simulink model "ForceBasedRollCenterVehicleModel"  (R2021b)
settings: Solver=VariableStepAuto  StartTime=0.0  StopTime=10.0  RelTol=1e-3
values from neighbouring files (symbols this model uses):
  AirDensity = 1.225    [PlanarModelWrapperScriptAttempt2.m]
  CoG = [(0.47-0.5)*Wheelbase, 0, 0.25]    [ForceBasedRollCenterModelWrapperScript.m]    (also in PlanarModelWrapperScriptAttempt2.m)
  CoP = [(0.4-0.5)*Wheelbase, 0, 0]    [PlanarModelWrapperScriptAttempt2.m]
  DragCoeff = 0.6    [PlanarModelWrapperScriptAttempt2.m]
  Front_Roll_Stiffness = 0    [ForceBasedRollCenterModelWrapperScript.m]
  Idx = 1    [3DOF Launch ControlHoosier_R25B_clean.mat]    (also in PlanarModelWrapperScriptAttempt2.m)
  Inclination = 1    [3DOF Launch ControlHoosier_R25B_clean.mat]    (also in PlanarModelWrapperScriptAttempt2.m)
  LiftCoeff = -1.9    [PlanarModelWrapperScriptAttempt2.m]
  Mass = 275    [ForceBasedRollCenterModelWrapperScript.m]    (also in PlanarModelWrapperScriptAttempt2.m)
  Model =     [3DOF Launch ControlHoosier_R25B_clean.mat]    (also in PlanarModelWrapperScriptAttempt2.m = struct( 'Pure', 'Pacejka', 'Combined', 'MNC' ))
  PercentFront = 0.5    [ForceBasedRollCenterModelWrapperScript.m]    (also in PlanarModelWrapperScriptAttempt2.m)
  PerLLT = 0.6    [PlanarModelWrapperScriptAttempt2.m]
  Pressure = 70    [3DOF Launch ControlHoosier_R25B_clean.mat]    (also in PlanarModelWrapperScriptAttempt2.m = 80)
  Rear_Roll_Stiffness = 0    [ForceBasedRollCenterModelWrapperScript.m]
  RefArea = 1.1    [PlanarModelWrapperScriptAttempt2.m]
  Roll_Dampening_Coeff_Front = 0    [ForceBasedRollCenterModelWrapperScript.m]
  Roll_Dampening_Coeff_Rear = 0    [ForceBasedRollCenterModelWrapperScript.m]
  Sprung_COG_Height = 0    [ForceBasedRollCenterModelWrapperScript.m]
  Tire =     [3DOF Launch ControlHoosier_R25B_clean.mat]
  TrackWidth = 1.22    [ForceBasedRollCenterModelWrapperScript.m]    (also in PlanarModelWrapperScriptAttempt2.m = 1.22*ones(1,2))
  TrackWidthTest = 1.22*ones(1,2)    [ForceBasedRollCenterModelWrapperScript.m]
  Wheelbase = 1.575    [ForceBasedRollCenterModelWrapperScript.m]    (also in PlanarModelWrapperScriptAttempt2.m)
  YawInertia = 130    [ForceBasedRollCenterModelWrapperScript.m]    (also in PlanarModelWrapperScriptAttempt2.m)
settings Model: Creator=jpchi  LastModifiedBy=jpchi

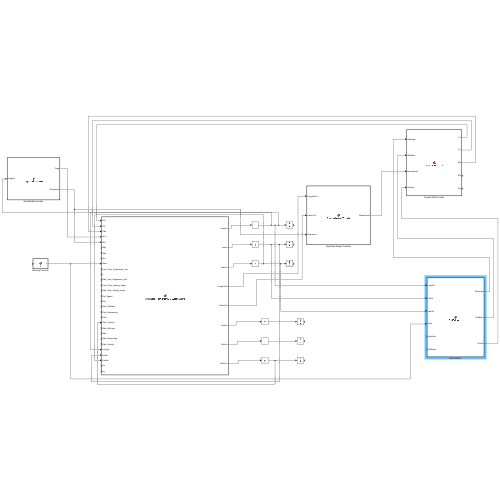
[thumbnail: Simulink's stored preview of the top-level diagram]
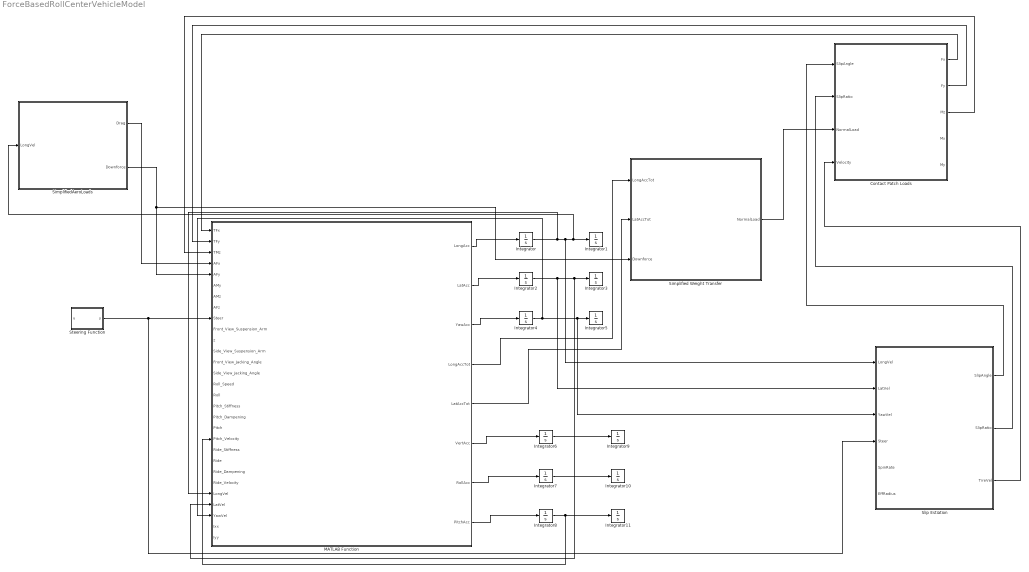
== system ForceBasedRollCenterVehicleModel ==
  Contact Patch Loads : MATLAB Function  TreatAsAtomicUnit=on
  Integrator{,1..11} (12 alike) : Integrator
  MATLAB Function : MATLAB Function  TreatAsAtomicUnit=on
  Simplified Weight Transfer : MATLAB Function  TreatAsAtomicUnit=on
  SimplifiedAeroLoads : MATLAB Function  TreatAsAtomicUnit=on
  Slip Estiation : MATLAB Function  TreatAsAtomicUnit=on
  Steering Function : MATLAB Function  TreatAsAtomicUnit=on
  wires:
  Steering Function/1(y) -> Slip Estiation/4(Steer), MATLAB Function/9(Steer)
  SimplifiedAeroLoads/2(Downforce) -> Simplified Weight Transfer/3(Downforce), MATLAB Function/5(AFy)
  SimplifiedAeroLoads/1(Drag) -> MATLAB Function/4(AFx)
  MATLAB Function/5(LatAccTot) -> Simplified Weight Transfer/2(LatAccTot)
  MATLAB Function/4(LongAccTot) -> Simplified Weight Transfer/1(LongAccTot)
  Simplified Weight Transfer/1(NormalLoad) -> Contact Patch Loads/3(NormalLoad)
  MATLAB Function/1(LongAcc) -> Integrator/1
  Integrator/1 -> MATLAB Function/25(LongVel), Slip Estiation/1(LongVel), SimplifiedAeroLoads/1(LongVel), Integrator1/1
  MATLAB Function/2(LatAcc) -> Integrator2/1
  Integrator2/1 -> Slip Estiation/2(LatVel), MATLAB Function/26(LatVel), Integrator3/1
  MATLAB Function/3(YawAcc) -> Integrator4/1
  Integrator4/1 -> MATLAB Function/27(YawVel), Slip Estiation/3(YawVel), Integrator5/1
  Slip Estiation/1(SlipAngle) -> Contact Patch Loads/1(SlipAngle)
  Slip Estiation/2(SlipRatio) -> Contact Patch Loads/2(SlipRatio)
  Slip Estiation/3(TireVel) -> Contact Patch Loads/4(Velocity)
  Contact Patch Loads/1(Fx) -> MATLAB Function/1(TFx)
  Contact Patch Loads/2(Fy) -> MATLAB Function/2(TFy)
  Contact Patch Loads/3(Mz) -> MATLAB Function/3(TMz)
  MATLAB Function/6(VertAcc) -> Integrator6/1
  MATLAB Function/7(RollAcc) -> Integrator7/1
  MATLAB Function/8(PitchAcc) -> Integrator8/1
  Integrator6/1 -> Integrator9/1
  Integrator7/1 -> Integrator10/1
  Integrator8/1 -> MATLAB Function/20(Pitch_Velocity), Integrator11/1

== matlab function ForceBasedRollCenterVehicleModel/SimplifiedAeroLoads ==
  data: LongVel input; Drag output; Downforce output; AirDensity parameter; RefArea parameter; DragCoeff parameter; LiftCoeff parameter
function [Drag, Downforce] = SimplifiedAeroLoads( LongVel, ...
    AirDensity, RefArea, DragCoeff, LiftCoeff)
%% SimplifiedWeightTransfer - Simplified Normal Loads
% Computes tire normal loads using simplified weight transfer and
% aerodynamic loading.
% 
% Inputs:
%   LongVel    - (n,1 numeric) Longitudinal Velocity {dot{x}}  [m/s]
%   AirDensity - (n,1 numeric) Air Density           {rho_air} [kg/m^3]
%   RefArea    - (n,1 numeric) Reference Area        {A}       [m^2]
%   DragCoeff  - (n,1 numeric) Drag Coefficient      {C_D}     [ ]
%   LiftCoeff  - (n,1 numeric) Lift Coefficient      {C_L}     [ ]
%
% Outputs:
%   Drag       - (n,1 numeric) Drag Force            {A_F_x}   [N]
%   Downforce  - (n,1 numeric) Downforce             {A_F_z}   [N]
%
% Notes:
%
% Author(s): 
% Blake Christierson (bechristierson@ucdavis.edu) [Sep 2018 - Jun 2021] 
% 
% Last Updated: 31-May-2021

%% Test Case
if nargin == 0
   LongVel = 15;
   
   AirDensity = 1.225;
   
   RefArea = 1.1;
   
   DragCoeff = 0.6;
   LiftCoeff = -1.9;
   
   [Drag, Downforce] = SimplifiedAeroLoads( LongVel, ...
    AirDensity, RefArea, DragCoeff, LiftCoeff ) %#ok<NOPRT>

    return
end

%% Computation
Drag      = 1/2 .* AirDensity .*  DragCoeff .* RefArea .* LongVel.^2;
Downforce = 1/2 .* AirDensity .* -LiftCoeff .* RefArea .* LongVel.^2;

end

== matlab function ForceBasedRollCenterVehicleModel/Slip Estiation ==
  data: LongVel input; SlipAngle output; LatVel input; YawVel input; Steer input; SpinRate input; EffRadius input; SlipRatio output; TireVel output; TirePos parameter
function [SlipAngle, SlipRatio, TireVel] = SlipEstimation( ...
    LongVel, LatVel, YawVel, Steer, SpinRate, EffRadius, TirePos)

%% SlipEstimation - Slip Angle and Slip Ratio Calculations
% Estimates tire slips and center velocity from chassis velocity and a
% handful of tire states.
% 
% Inputs:
%   LongVel   - (1,1 numeric) Longitudinal Velocity {x_dot}   [m/s]
%   LatVel    - (1,1 numeric) Lateral Velocity      {y_dot}   [m/s]
%   YawVel    - (1,1 numeric) Yaw Rate              {psi_dot} [rad/s]
%   TirePos   - (n,3 numeric) [x,y,0] Tire Position {p}       [m]
%   Steer     - (n,1 numeric) Tire Steer Angle      {delta}   [deg]
%   SpinRate  - (n,1 numeric) Tire Spin Rate        {omega}   [rad/s]
%   EffRadius - (n,1 numeric) Tire Effective Radius {r_e}     [m]
% 
% Outputs:
%   SlipAngle - (n,1 numeric) Tire Slip Angle      {alpha} [deg]
%   SlipRatio - (n,1 numeric) Tire Slip Ratio      {kappa} [ ]
%   TireVel   - (n,1 numeric) Tire Center Velocity {v_c}   [m/s]
%
% Notes:
%   Typically n=4; however, may be vectorized by stacking rows.
%
% Author(s): 
% Blake Christierson (bechristierson@ucdavis.edu) [Sep 2018 - Jun 2021] 
%
% Last Updated: 1-Apr-2021

%% Test Cases
if nargin == 0
    LongVel = 10;
    LatVel = 2;
    YawVel = 0.1;
    TirePos = [ 0.84  0.66 0; ...
                0.84 -0.66 0; ...
               -0.67  0.66 0; ...
               -0.67 -0.66 0];
    
    Steer = [25; 20; -0.5; 0.5];
    
    SpinRate = 100 .* ones(4,1);
    EffRadius = 0.19 .* ones(4,1);
    
    [SlipAngle, SlipRatio, TireVel] = SlipEstimation( ...
        LongVel, LatVel, YawVel, TirePos, Steer, SpinRate, EffRadius);

    fprintf('Executing SlipEstimation() Test Cases: \n');
    for i = 1:numel(SlipAngle)
        fprintf('   Instance %i: \n', i);
        fprintf('      alpha = %5.2f [deg] \n', SlipAngle(i));
        fprintf('      kappa = %5.2f [ ] \n', SlipRatio(i));
        fprintf('      v_c   = %5.2f [m/s] \n', TireVel(i));
    end
    
    return;
end

%% Computation
%%% Number of Evaluations
n = numel(Steer);

%%% Tire Center Velocities
TireVel = zeros(n,3);
for i = 1:n
    TireVel(i,:) = [LongVel; LatVel; 0] + cross( [0; 0; YawVel], TirePos(i,:)' );
end

%%% Slip Angle
SlipAngle = atan2d( TireVel(:,2), TireVel(:,1) ) - Steer;

%%% Slip Ratio
SlipRatio = ( SpinRate .* EffRadius ) ./ ( norm(TireVel,2) .* cosd( SlipAngle ) ) - 1;

== matlab function ForceBasedRollCenterVehicleModel/Contact Patch Loads ==
  data: Fx output; SlipAngle input; SlipRatio input; NormalLoad input; Velocity input; Fy output; Mz output; Mx output; My output; Tire parameter; Pressure parameter; Inclination parameter; Idx parameter; Model parameter
function [Fx, Fy, Mz, Mx, My] = ContactPatchLoads( SlipAngle, SlipRatio, ...
    NormalLoad, Velocity, ...
    Tire, ...
Pressure, Inclination, Idx, Model)
%% ContactPatchLoads - Tire Load Evaluation
% This script evaluates a Pacejka contact patch tire model using the
% formatted by TireModelFittingMain(). 
% 
% Inputs:
%   Tire          - (struct)      Pacejka Parameters
%   SlipAngle     - (n,1 numeric) Slip Angle          {alpha} [deg]
%   SlipRatio     - (n,1 numeric) Slip Ratio          {kappa} [ ]
%   NormalLoad    - (n,1 numeric) Normal Load         {F_z}   [N]
%   Pressure      - (n,1 numeric) Inflation Pressure  {P_i}   [kPa]
%   Inclination   - (n,1 numeric) Inclination Angle   {gamma} [deg]
%   Velocity      - (n,1 numeric) Center Velocity     {v_c}   [m/s]
%   Idx           - (n,1 numeric) Corner Idx          {1-4}   [ ]
%   Model         - (struct)      Fidelity Choices 
%       .Pure     - (char)        Pure Slip Model     {'Linear', 'Pacejka'}
%       .Combined - (char)        Combined Slip Model {'Pure', 'MNC', 'Pacejka'}
%
% Outputs:
%   Fx - (n,1 numeric) Longitudinal (Tractive) Force {F_x} [N]
%   Fy - (n,1 numeric) Lateral Force                 {F_y} [N]
%   Mz - (n,1 numeric) Aligning Moment               {M_z} [N-m]
%   Mx - (n,1 numeric) Overturning Moment            {M_x} [N-m]
%   My - (n,1 numeric) Rolling Resistance            {M_y} [N-m]
%
% Notes:
%   Pacejka combined slip model is not currently implemented (4/2/21) and
%   when the model does become available the model compatibility checks
%   should be reformatted.
%
% Author(s): 
% Blake Christierson (bechristierson@ucdavis.edu) [Sep 2018 - Jun 2021] 
% Carlos Lopez       (calopez@ucdavis.edu       ) [Jan 2019 -         ]
% Leonardo Howard    (leohoward@ucdavis.edu     ) [Jan 2021 -         ]
% Tristan Pham       (atlpham@ucdavis.edu       ) [Jan 2021 -         ]
% 
% Last Updated: 11-Nov-2021

%% Test Case
if nargin == 0
    warning('Executing SlipEstimation() Test Case')
    
    addpath( genpath( fileparts( which( 'ContactPatchLoads.m' ) ) ) );
    %load('Models\TestTire.mat'); %#ok<LOAD> missing Tire.Pacejka.p.P.Mx
    load('Hoosier_R25B_18x75-10x7.mat');
    %load('Hoosier_R25B_16x75-10x7.mat');
    %load('Tire.mat');
    
    %%% Nominal Test Case Conditions
    Pressure    = 70;
    Inclination = 1;
    Velocity    = 10;
    Idx         = 1;
    Model       = struct( 'Pure', 'Pacejka', 'Combined', 'MNC' );
    
    %%% Slip-Load Plots 
    SlipRatio = linspace(- 1, 1,51);
    SlipAngle = linspace(-20,20,51);
    
    NormalLoad  = 0:100:2000;
        
    [~         , SlipRatio] = meshgrid( NormalLoad, SlipRatio );
    [NormalLoad, SlipAngle] = meshgrid( NormalLoad, SlipAngle );
    
    [Fx, Fy, Mz, Mx, My] = ContactPatchLoads( Tire, ...
        SlipAngle, SlipRatio, ...
        NormalLoad, Pressure, Inclination, Velocity, ...
        Idx, Model );
     
    figure
    sgtitle( {'Slip-Load Surfaces', ...
        ['$P_{i} ='  , num2str(Pressure)   , '$ [$kPa$],' ...
          '$\gamma = ', num2str(Inclination), '$ [$deg$]']} )
      
    subplot(3,2,1)
    surf( SlipRatio, NormalLoad, Fx )
    xlabel( '$\kappa$ [ ]' )
    ylabel( '$F_{z}$ [$N$]' )
    zlabel( '$F_{x}$ [$N$]' )
    title( 'Longitudinal Force' )
    
    subplot(3,2,2)
    surf( SlipAngle, NormalLoad, Fy )
    xlabel( '$\alpha$ [$deg$]' )
    ylabel( '$F_{z}$ [$N$]' )
    zlabel( '$F_{y}$ [$N$]' )
    title( 'Lateral Force' )
    
    subplot(3,2,3)
    surf( SlipAngle, NormalLoad, Mz )
    xlabel( '$\alpha$ [$deg$]' )
    ylabel( '$F_{z}$ [$N$]' )
    zlabel( '$M_{z}$ [$Nm$]' )
    title( 'Aligning Moment' )
    
    subplot(3,2,4)
    surf( SlipAngle, NormalLoad, Mx )
    xlabel( '$\alpha$ [$deg$]' )
    ylabel( '$F_{z}$ [$N$]' )
    zlabel( '$M_{x}$ [$Nm$]' )
    title( 'Overturning Moment' )
    
    subplot(3,2,5)
    surf( SlipRatio, NormalLoad, My )
    xlabel( '$\kappa$ [ ]' )
    ylabel( '$F_{z}$ [$N$]' )
    zlabel( '$M_{y}$ [$Nm$]' )
    title( 'Rolling Resistance' )
      
    %%% Friction Ellipse Plotting
    SlipRatio = linspace(- 1, 1,51);
    SlipAngle = linspace(-20,20,51);
    
    [SlipRatio, SlipAngle] = meshgrid( SlipRatio, SlipAngle );
    
    NormalLoad = 700;
    
    [Fx, Fy, ~, ~, ~] = ContactPatchLoads( Tire, ...
        SlipAngle, SlipRatio, ...
        NormalLoad, Pressure, Inclination, Velocity, ...
        Idx, Model );

    ColorMap = colormap( 'parula' );
    figure
    for i = 1 : size( SlipAngle, 1)
        plot( Fy(i,:), Fx(i,:), 'Color', ...
            ColorMap( round( (SlipAngle(i,1)-SlipAngle(1)) .* ...
                (length(ColorMap)-1) ./ diff( SlipAngle([1 end]) )) + 1, : ) ); hold on;
    end
    
    for j = 1 : size( SlipRatio, 2)
        plot( Fy(:,j), Fx(:,j), 'Color', ...
            ColorMap( round( (SlipRatio(1,j)-SlipRatio(1)) .* ...
                (length(ColorMap)-1) ./ diff( SlipRatio([1 end]) )) + 1, : ) );
    end
    
    xlabel( 'Lateral Force, $F_{y}$ [$N$]' ); 
    ylabel( 'Longitudinal Force, $F_{x}$ [$N$]' );
    title( 'Friction Ellipse' )
    
    %%% Inclination Sensitivity
    Inclination = -3:0.05:3;
    
    SlipRatio = linspace(- 1, 1,51);
    SlipAngle = linspace(-20,20,51);
    
    [~          , SlipRatio] = meshgrid( Inclination, SlipRatio );
    [Inclination, SlipAngle] = meshgrid( Inclination, SlipAngle );
    
    [Fx, Fy, ~, ~, ~] = ContactPatchLoads( Tire, ...
        SlipAngle, SlipRatio, ...
        NormalLoad, Pressure, Inclination, Velocity, ...
        Idx, Model );
    
    figure
    plot( Inclination(1,:), max(abs(Fx),[],1)./max(abs(Fx),[],'all') ); hold on;
    plot( Inclination(1,:), max(abs(Fy),[],1)./max(abs(Fy),[],'all') )
    
    xlabel( 'Inclination, $\gamma$ [$deg$]' )
    ylabel( 'Normalized Grip' )
    title( 'Inclination Sensitivity')
    legend( '$F_{x}$', '$F_{y}$' )
    
    %%% Single Evaluation
    Inclination = 1;
    SlipAngle = 5;
    SlipRatio = 0.03;
    
    [Fx, Fy, Mz, Mx, My] = ContactPatchLoads( Tire, ...
        SlipAngle, SlipRatio, ...
        NormalLoad, Pressure, Inclination, Velocity, ...
        Idx, Model );
    
    return;
end

%% Model Compatibility Check
if ~ismember(Model.Pure, {'Linear', 'Pacejka'})
    error('Please choose either ''Linear'' or ''Pacejka'' for the pure slip model')
elseif ~ismember(Model.Combined, {'Pure', 'MNC'})
    if strcmp(Model.Combined, 'Pacejka')
        error('The Pacejka combined slip model is not implemented (4/2/21)')
    else
        error('Please choose either ''Pure'' or ''MNC'' for the combined slip model')
    end
end

%% Main Evaluation
%%% Slip Angle Conversion
SlipAngle = deg2rad(SlipAngle);

%%% Left-Right Side Orientation Manipulation
% Ensures model conicity & ply-steer are symmetric to prevent drift
SlipAngle = SlipAngle .* (-1).^(mod(Idx+1,2));
Inclination   = Inclination   .* (-1).^(mod(Idx+1,2));

%%% Nondimensional Load & Pressure
dFz = (NormalLoad - Tire.Pacejka.Fzo) ./ Tire.Pacejka.Fzo;
dPi = (Pressure - Tire.Pacejka.Pio) ./ Tire.Pacejka.Pio;

%%% Evaluate Pure Slip Forces & Aligning Moment
[Fx0, Kxk, Kappa0] = EvaluateFx0( Tire, SlipAngle, SlipRatio, ...
    NormalLoad, dFz, Pressure, dPi, Inclination, Velocity, Idx, Model ); 

[Fy0, By, Cy, Kya, Hy, Vy, Alpha0] = EvaluateFy0( Tire, SlipAngle, SlipRatio, ...
    NormalLoad, dFz, Pressure, dPi, Inclination, Velocity, Idx, Model ); 
    
[Fyo, ~, ~, ~, ~, ~, Alphao] = EvaluateFy0( Tire, SlipAngle, SlipRatio, ...
    NormalLoad, dFz, Pressure, dPi, 0  , Velocity, Idx, Model );

[Mz0, Bt, Ct, Dt, Et, Ht, Br, Cr, Dr, Hf] = EvaluateMz0( Tire, SlipAngle, SlipRatio, ...
    NormalLoad, dFz, Pressure, dPi, Inclination, Velocity, Idx, Model, ...
    Fyo, By, Cy, Kya, Hy, Vy );

%%% Combined Slip Force Models 
switch Model.Combined
    case 'Pure' % Pure Slip Only Model
        Fx  = Fx0;
        Fy  = Fy0;   

    case 'MNC' % Modified-Nicolas-Comstock Combined Slip Model
        [Fx, Fy ]  = MNCCombinedSlipForces( Tire, ...
            SlipAngle, SlipRatio, Fx0, Fy0, Kxk, Kya, Kappa0, Alpha0 );
        [~ , Fyp]  = MNCCombinedSlipForces( Tire, ...
            SlipAngle, SlipRatio, Fx0, Fyo, Kxk, Kya, Kappa0, Alphao );

    case 'MF6_1' % Combined Slip Pacejka MF6.1 Model
        % Not Implemented
end

%%% Evaluate Combined Slip Aligning Moment (Mz)
if strcmpi( Model.Combined, 'Pure' )
    Mz = Mz0;
else
    Mz = EvaluateMz( Tire, SlipAngle, SlipRatio, ...
        NormalLoad, dFz, Pressure, dPi, Inclination, Velocity, Idx, Model, ...
        Fx, Fy, Fyp, Kxk, Kya, Bt, Ct, Dt, Et, Ht, Br, Cr, Dr, Hf );
end

%%% Evaluate Moment & Rolling Resistance
Mx = EvaluateMx( Tire, SlipAngle, SlipRatio, ...
    NormalLoad, dFz, Pressure, dPi, Inclination, Velocity, Idx, Model, Fy );

My = EvaluateMy( Tire, SlipAngle, SlipRatio, ...
    NormalLoad, dFz, Pressure, dPi, Inclination, Velocity, Idx, Model, Fx );

%%% Pure Slip Longitudinal Force Evaluation (Fx0)
function [Fx0, Kxk, Kappa0] = ...
        EvaluateFx0( Tire, ~, Kappa, Fz, dFz, ~, dPi, Inc, ~, ~, Model )
    
    % Evaluate P6 Pacejka
    Cx = Tire.Pacejka.p.C.x(1) .* Tire.Pacejka.L.C.x;

    Dx = (Tire.Pacejka.p.D.x(1) + Tire.Pacejka.p.D.x(2).*dFz) .* ...
         (1 + Tire.Pacejka.p.P.x(3).*dPi + Tire.Pacejka.p.P.x(4).*dPi.^2) .* ...
         (1 - Tire.Pacejka.p.D.x(3).*Inc.^2).*Fz .* Tire.Pacejka.L.mu.x;

    Ex = ( Tire.Pacejka.p.E.x(1) + Tire.Pacejka.p.E.x(2).*dFz ...
        + Tire.Pacejka.p.E.x(3).*dFz.^2 ) .* ( 1 - Tire.Pacejka.p.E.x(4).*sign(Kappa) ) .* ...
        Tire.Pacejka.L.E.x;

    Kxk = Fz.*(Tire.Pacejka.p.K.x(1) + Tire.Pacejka.p.K.x(2).*dFz ) .* ...
        exp( Tire.Pacejka.p.K.x(3) .* dFz ) .* ...
        (1 + Tire.Pacejka.p.P.x(1).*dPi + Tire.Pacejka.p.P.x(2).*dPi.^2) .* ...
        Tire.Pacejka.L.K.x.k;

    Bx = Kxk ./ ( Cx.*Dx );

    Vx = Fz.*(Tire.Pacejka.p.V.x(1) + Tire.Pacejka.p.V.x(2).*dFz ) .* ...
        Tire.Pacejka.L.V.x;

    Hx = (Tire.Pacejka.p.H.x(1) + Tire.Pacejka.p.H.x(2).*dFz) .* ...
        Tire.Pacejka.L.H.x;

    % Evaluate Longitudinal Force​
    switch Model.Pure
        case 'Linear'
            Fx0 = Kxk .* Kappa;
        case 'Pacejka'
            Fx0 = Dx .* sin( Cx .* atan( (1-Ex) .* Bx.*(Kappa + Hx) + ...
                Ex.*atan( Bx.*(Kappa + Hx) ) ) ) + Vx;
    end

    % Evaluate Null Slip Ratio
    if strcmpi( Model.Combined, 'MNC' )
        Kappa0 = -Vx ./ Kxk - Hx;
        Kappa0(isnan(Kappa0)) = 0; % Can use smoothing in future
    else
        Kappa0 = [];
    end
end

%%% Pure Slip Lateral Force Evaluation (Fy0)
function [Fy0, By, Cy, Kya, Hy, Vy, Alpha0] = ...
        EvaluateFy0( Tire, Alpha, ~, Fz, dFz, ~, dPi, Inc, ~, i, Model )            
    
    % Evaluate P6 Pacejka
    Cy = Tire.Pacejka.p.C.y(1);

    Dy = (Tire.Pacejka.p.D.y(1) + Tire.Pacejka.p.D.y(2).*dFz) .* ...
         (1 + Tire.Pacejka.p.P.y(3).*dPi + Tire.Pacejka.p.P.y(4).*dPi.^2) .* ...
         (1 - Tire.Pacejka.p.D.y(3).*Inc.^2).*Fz;

    Kya = Tire.Pacejka.p.K.y(1) .* Tire.Pacejka.Fzo .* ( 1 + Tire.Pacejka.p.P.y(1).*dPi ) .* ...
        ( 1 - Tire.Pacejka.p.K.y(3).*abs(Inc) ) .* sin( Tire.Pacejka.p.K.y(4) .* ...
        atan( (Fz./Tire.Pacejka.Fzo) ./ ...
        ( ( Tire.Pacejka.p.K.y(2) + Tire.Pacejka.p.K.y(5).*Inc.^2 ) .* ...
        ( 1 + Tire.Pacejka.p.P.y(2).*dPi ) ) ) );

    Kyg0 = Fz.*(Tire.Pacejka.p.K.y(6) + Tire.Pacejka.p.K.y(7).*dFz ) .* ...
        (1 + Tire.Pacejka.p.P.y(5).*dPi );

    By = Kya ./ ( Cy.*Dy );

    Vyg = Fz.*(Tire.Pacejka.p.V.y(3) + Tire.Pacejka.p.V.y(4).*dFz ).*Inc;

    Vy = Fz.*(Tire.Pacejka.p.V.y(1) + Tire.Pacejka.p.V.y(2).*dFz ) + Vyg;

    Hy = (Tire.Pacejka.p.H.y(1) + Tire.Pacejka.p.H.y(2).*dFz ) .* (Kyg0.*Inc - Vyg ) ./ Kya;

    Ey = ( Tire.Pacejka.p.E.y(1) + Tire.Pacejka.p.E.y(2).*dFz ) .* ...
        ( 1 + Tire.Pacejka.p.E.y(5).*Inc.^2 - ...
        ( Tire.Pacejka.p.E.y(3) + Tire.Pacejka.p.E.y(4).*Inc ).*sign(Alpha + Hy) );

    % Evaluate Lateral Force
    switch Model.Pure
        case 'Linear'
            Fy0 = Kya .* Alpha;
        case 'Pacejka'
            Fy0 = (Dy .* sin( Cy .* atan( (1-Ey) .* By.*( Alpha + Hy ) + ...
                Ey .* atan( By.*( Alpha + Hy ) ) ) ) + Vy) .* (-1).^(mod(i+1,2));
    end

    % Evaluate Null Slip Angle
    if strcmpi( Model.Combined, 'MNC' )
        Alpha0 = -Vy ./ Kya - Hy;
        Alpha0(isnan(Alpha0)) = 0;
    else
        Alpha0 = [];
    end
end

%%% Evaluate Pure Slip Aligning Moment (Mz0)
function [Mz0, Bt, Ct, Dt, Et, Ht, Br, Cr, Dr, Hf] = ...
        EvaluateMz0( Tire, Alpha, ~, Fz, dFz, ~, dPi, Inc, ~, i, ~, ...
            Fyo, By, Cy, Kya, Hy, Vy )
    
    % Evaluate P6 Pacejka
    Bt = (Tire.Pacejka.q.B.z(1) + Tire.Pacejka.q.B.z(2).*dFz + ...
        Tire.Pacejka.q.B.z(3).*dFz.^2) .* ...
        (1 + Tire.Pacejka.q.B.z(5).*abs(Inc) + ...
        Tire.Pacejka.q.B.z(6).*Inc.^2);

    Ct = Tire.Pacejka.q.C.z(1);

    Dt = (Tire.Pacejka.Ro ./ Tire.Pacejka.Fzo) .* ...
        ( Tire.Pacejka.q.D.z(5) .* (Tire.Pacejka.Fzo ./ Tire.Pacejka.Ro) + ...
        Tire.Pacejka.q.D.z(1).*Fz + Tire.Pacejka.q.D.z(2).*Fz.*dFz ) .* ...
        ( 1 - Tire.Pacejka.p.P.z(1).*dPi ) .* ...
        ( 1 + Tire.Pacejka.q.D.z(3).*abs(Inc) + ...
        Tire.Pacejka.q.D.z(4).*Inc.^2 );

    Ht = Tire.Pacejka.q.H.z(1) + ...
        Tire.Pacejka.q.H.z(2).*dFz + (Tire.Pacejka.q.H.z(3) + ...
        Tire.Pacejka.q.H.z(4).*dFz).*Inc;

    Et = (Tire.Pacejka.q.E.z(1) + Tire.Pacejka.q.E.z(2).*dFz + ...
        Tire.Pacejka.q.E.z(3).*dFz.^2) .* ...
        (1 + (Tire.Pacejka.q.E.z(4) + Tire.Pacejka.q.E.z(5).*Inc).*(2/pi).* ...
        atan( Bt .* Ct .* (Alpha+Ht) ) );

    Br = Tire.Pacejka.q.B.z(10) .* By .* Cy;

    Cr = 1;

    Dr = Tire.Pacejka.Ro .* Fz .* ( ( Tire.Pacejka.q.D.z(6) + ...
        Tire.Pacejka.q.D.z(7).*dFz ) + ...
        ( ( Tire.Pacejka.q.D.z(8) + Tire.Pacejka.q.D.z(9).*dFz ) .* ...
        ( 1 + Tire.Pacejka.p.P.z(2).*dPi ) + ...
        ( Tire.Pacejka.q.D.z(10) + Tire.Pacejka.q.D.z(11).*dFz ) .* ...
        abs(Inc) ).*Inc ) .* cos( Alpha );

    Hf = Hy + Vy ./ Kya;

    % Evaluate Trail Function
    t0 = Dt.*cos( Ct.*atan( (1-Et).*(Bt.*(Alpha + Ht)) + ...
        Et.*atan( Bt.*(Alpha + Ht) ) ) ) .* cos( Alpha ) ;

    % Evaluate Residual Aligning Moment
    Mzro = Dr .* cos( Cr.*atan( Br.*(Alpha + Hf) ) ).* cos( Alpha );

    % Evaluate Pure Slip Aligning Moment (Mz0)
    Mz0 = (-t0 .* Fyo .* (-1).^(mod(i+1,2)) + Mzro) .* (-1).^(mod(i+1,2));
end

%%% Modified-Nicolas Comstock Combined Slip Forces
function [Fx, Fy] = MNCCombinedSlipForces( ~, Alpha, Kappa, Fx0, Fy0, Kxk, Kya, Kappa0, Alpha0 )
    Fx = abs(Fx0 .* Fy0 ./ sqrt( (Kappa - Kappa0).^2 .* Fy0.^2 + Fx0.^2 .* tan(Alpha - Alpha0).^2 ) .* ...
        sqrt( (Kappa - Kappa0).^2 .* Kya.^2 + (1 - abs(Kappa - Kappa0)).^2 .* cos(Alpha - Alpha0).^2 .* Fx0.^2 ) ./ Kya) .* sign(Fx0);

    Fy = abs( Fx0 .* Fy0 ./ sqrt( (Kappa - Kappa0).^2 .* Fy0.^2 + Fx0.^2 .* tan(Alpha - Alpha0).^2 ) .* ...
        sqrt( (1 - abs(Kappa - Kappa0)).^2 .* cos(Alpha - Alpha0).^2 .* Fy0.^2 + sin(Alpha - Alpha0).^2 .* Kxk.^2 ) ./ ...
        ( Kxk .* cos(Alpha - Alpha0)) ) .* sign(Fy0);
end

%%% Evaluate Combined Slip Aligning Moment (Mz)
function Mz = EvaluateMz( Tire, Alpha, Kappa, ~, dFz, ~, ~, Inc, ~, i, ~, ...
    Fx, Fy, Fyp, Kxk, Kya, Bt, Ct, Dt, Et, Ht, Br, Cr, Dr, Hf )
    
    % Equivalent Slips
    Alphat = (Alpha + (-1).^(mod(i+1,2)).*Ht );
    Alphar = (Alpha + (-1).^(mod(i+1,2)).*Hf );

    Alphateq = sqrt( Alphat.^2 + (Kxk./Kya).^2 .* Kappa.^2 ) .* sign( Alphat );
    Alphareq = sqrt( Alphar.^2 + (Kxk./Kya).^2 .* Kappa.^2 ) .* sign( Alphar );

    % Evaluate Trail Function
    t = Dt.*cos( Ct.*atan( (1-Et).*(Bt.*Alphateq) + ...
        Et.*atan(Bt.*Alphateq) ) ) .* cos( Alpha );

    % Evaluate Scrub Function
    s = Tire.Pacejka.Ro .* (Tire.Pacejka.s.s.z(1) + ...
        Tire.Pacejka.s.s.z(2) .* (Fy./Tire.Pacejka.Fzo) + ...
        (Tire.Pacejka.s.s.z(3) + Tire.Pacejka.s.s.z(4) .* dFz) .* Inc );

    % Evaluate Residual Aligning Moment
    Mzr = Dr .* cos( Cr.*atan( Br.*(Alphareq) ) ) .* cos( Alpha );

    % Evaluate Pure Slip Aligning Moment (Mz0)
    Mz = -t .* Fyp + Mzr + s .* Fx;
end

%%% Evaluate Overturning Moment
function Mx = EvaluateMx( Tire, ~, ~, Fz, ~, ~, dPi, Inc, ~, ~, ~, Fy )
    Mx = Tire.Pacejka.Ro .* Fz .* ( Tire.Pacejka.q.s.x(1) - ...
        Tire.Pacejka.q.s.x(2) .* Inc .* ( 1 + Tire.Pacejka.p.P.Mx(1).*dPi ) + ...
        Tire.Pacejka.q.s.x(3) .* Fy ./ Tire.Pacejka.Fzo + ...
        Tire.Pacejka.q.s.x(4) .* cos( Tire.Pacejka.q.s.x(5) .* ...
        ( atan( (Tire.Pacejka.q.s.x(6) .* Fz ./ Tire.Pacejka.Fzo) ) ).^2 ) .* ...
        sin( Tire.Pacejka.q.s.x(7) .* Inc + Tire.Pacejka.q.s.x(8) .* ...
        atan( Tire.Pacejka.q.s.x(9) .* Fy ./ Tire.Pacejka.Fzo ) ) + ...
        Tire.Pacejka.q.s.x(10) .* atan( Tire.Pacejka.q.s.x(11) .* Fz ./ Tire.Pacejka.Fzo ) .* Inc );
end

%%% Evaluate Rolling Resistance
function My = EvaluateMy( Tire, ~, Kappa, Fz, ~, Pi, ~, ~, V, ~, ~, Fx )
    Re = Tire.Radius.Effective( Kappa, Fz, Pi );
    Rl = Tire.Radius.Loaded( Fz, Pi );
    
    My = Fx .* (Re - Rl) + Fz .* Re .* ( Tire.Pacejka.q.s.y(1) + ...
        Tire.Pacejka.q.s.y(3) .* (V ./ Tire.Pacejka.Vo) + ...
        Tire.Pacejka.q.s.y(4) .* (V ./ Tire.Pacejka.Vo).^4 );
end

end

== matlab function ForceBasedRollCenterVehicleModel/Steering Function ==
  data: u input; y output
function y = fcn(u)

y = u;

== matlab function ForceBasedRollCenterVehicleModel/Simplified Weight Transfer ==
  data: LongAccTot input; NormalLoad output; LatAccTot input; Wheelbase parameter; Downforce input; TrackWidth parameter; Mass parameter; CoG parameter; CoP parameter; PerLLT parameter
function NormalLoad  = SimplifiedWeightTransfer( LongAccTot, LatAccTot, ...
        Wheelbase, Downforce, TrackWidth, Mass, CoG, CoP, PerLLT) 
%% SimplifiedWeightTransfer - Simplified Normal Loads
% Computes tire normal loads using simplified weight transfer and
% aerodynamic loading.
% 
% Inputs:
%   LongAccTot - (n,1 numeric) Total Longitudinal Acceleration     {a_x}   [m/s^2]
%   LatAccTot  - (n,1 numeric) Total Lateral Acceleration          {a_y}   [m/s^2]
%   Wheelbase  - (n,1 numeric) Wheelbase                           {L}     [m]
%   TrackWidth - (n,2 numeric) Track Width                         {t_w}   [m]
%   Mass       - (n,1 numeric) Total Vehicle Mass                  {m}     [kg]
%   CoG        - (n,3 numeric) Center of Gravity                   {CoG}   [m]
%   Downforce  - (n,1 numeric) Aerodynamic Downforce               {A_F_z} [N]
%   CoP        - (n,3 numeric) Center of Pressure                  {CoP}   [m]
%   PerLLT     - (n,1 numeric) Percent Front Lateral Load Transfer {%_LLT} [ ]
%
% Outputs:
%   NormalLoad - (n,4 numeric) Tire Normal Loads                   {T_F_z} [N]
%
% Notes:
%
% Author(s): 
% Blake Christierson (bechristierson@ucdavis.edu) [Sep 2018 - Jun 2021] 
% 
% Last Updated: 30-May-2021

%% Test Case
if nargin == 0
    LongAccTot = 0; %-0.5 .* 9.81;
    LatAccTot  =  0.7 .* 9.81;
    
    Wheelbase = 1.575;
    TrackWidth = [1.22, 1.23];
    
    Mass = 275;
    CoG  = [(0.47-0.5)*Wheelbase, 0, 0.25];
    
    Downforce = 200;
    CoP  = [(0.4-0.5)*Wheelbase, 0, 0];
    
    PerLLT = 0.6;
    
    [NormalLoad] = SimplifiedWeightTransfer( LongAccTot, LatAccTot, ...
        Wheelbase, TrackWidth, Mass, CoG, Downforce, CoP, PerLLT ) %#ok<NOPRT>
    
    return
end

%% Computation
NormalLoad = zeros( [size( LongAccTot ), 4] );

%%% Total Weight Transfer
dFzx = Mass .* LongAccTot .* CoG(:,3) ./ Wheelbase;
dFzy = Mass .* LatAccTot  .* CoG(:,3) ./ mean(TrackWidth, 2);

%%% Static Wheel Loads
MassBal = (CoG(:,1) + Wheelbase./2) ./ Wheelbase;
AeroBal = (CoP(:,1) + Wheelbase./2) ./ Wheelbase;

NormalLoad(:,1:2) = (MassBal .* Mass .* 9.81 + AeroBal .* Downforce) / 2;
NormalLoad(:,3:4) = ((1-MassBal) .* Mass .* 9.81 + (1-AeroBal) .* Downforce) / 2;

%%% Dynamic Wheel Loads
NormalLoad(:,1) = NormalLoad(:,1) + (-0.5.*dFzx - PerLLT    .*dFzy)/2;
NormalLoad(:,2) = NormalLoad(:,2) + (-0.5.*dFzx + PerLLT    .*dFzy)/2;
NormalLoad(:,3) = NormalLoad(:,3) + ( 0.5.*dFzx - (1-PerLLT).*dFzy)/2;
NormalLoad(:,4) = NormalLoad(:,4) + ( 0.5.*dFzx + (1-PerLLT).*dFzy)/2;

end

== matlab function ForceBasedRollCenterVehicleModel/MATLAB Function ==
  data: TFx input; LongAcc output; TFy input; TMz input; AFx input; AFy input; AMy input; AMz input; AFz input; Steer input; Front_View_Suspension_Arm input; z input; Side_View_Suspension_Arm input; Front_View_Jacking_Angle input; Side_View_Jacking_Angle input; Roll_Speed input; Roll input; Pitch_Stiffness input; Pitch_Dampening input; Pitch input; Pitch_Velocity input; Ride_Stiffness input; Ride input; Ride_Dampening input; Ride_Velocity input; LongVel input; LatVel input; YawVel input; Ixx input; Iyy input; LatAcc output; YawAcc output; LongAccTot output; LatAccTot output; VertAcc output; RollAcc output; PitchAcc output; Wheelbase parameter; TrackWidth parameter; PercentFront parameter; Mass parameter; CoG parameter; Sprung_COG_Height parameter; YawInertia parameter; TrackWidthTest parameter; Front_Roll_Stiffness parameter; Rear_Roll_Stiffness parameter; Roll_Dampening_Coeff_Front parameter; Roll_Dampening_Coeff_Rear parameter
function [LongAcc, LatAcc, YawAcc, LongAccTot, LatAccTot, VertAcc, RollAcc, PitchAcc] = ...
    ForceBasedRollCenter6DOFAccelerations( TFx, TFy, TMz, AFx, AFy, AMy, AMz, AFz, ...       % Loads
        Steer, Front_View_Suspension_Arm, z, Side_View_Suspension_Arm, Front_View_Jacking_Angle, ...
        Side_View_Jacking_Angle, ...
        Roll_Speed, Roll, ...
        Pitch_Stiffness, Pitch_Dampening, Pitch, Pitch_Velocity, ...
        Ride_Stiffness, Ride, Ride_Dampening, Ride_Velocity,...
        LongVel, LatVel, YawVel, Ixx, Iyy, Wheelbase, TrackWidth, PercentFront, ...                      % Geometry                                                  % Velocities
Mass, CoG, Sprung_COG_Height, ...                                       % Inertia
YawInertia, TrackWidthTest, Front_Roll_Stiffness, Rear_Roll_Stiffness, Roll_Dampening_Coeff_Front, ...
Roll_Dampening_Coeff_Rear)
%% FroceBasedRollCenter6DOFAccelerations - Force Based Roll Center Accelerations
% Computes force based roll center accelerations for a 6DOF full track chassis model
% https://www.overleaf.com/project/5e73ad44ea180c00018cb332 (Section ?)
%
% Inputs:
%   TFx        - (n,4 numeric) Tire Longitudinal Force {T_F_y}    [N]
%   TFy        - (n,4 numeric) Tire Lateral Force      {T_F_y}    [N]
%   TMz        - (n,4 numeric) Tire Aligning Moment    {T_M_z}    [N-m]
%   AFx        - (n,1 numeric) Aerodynamic Drag Force  {A_F_x}    [N]
%   AFy        - (n,1 numeric) Aerodynamic Side Force  {A_F_y}    [N]
%   AMz        - (n,1 numeric) Aerodynamic Yaw Moment  {A_M_z}    [N-m]
%   Wheelbase  - (n,1 numeric) Wheelbase               {L}        [m]
%   TrackWidth - (n,2 numeric) Track Width             {t_w}      [m]
%   Steer      - (n,4 numeric) Tire Steer Angle        {delta}    [deg]
%   Mass       - (n,1 numeric) Total Vehicle Mass      {m}        [kg]
%   YawInertia - (n,1 numeric) Vehicle Yaw Inertia     {I_zz}     [kg-m^2]
%   CoG        - (n,3 numeric) Center of Gravity       {CoG}      [m]
%   LongVel    - (n,1 numeric) Longitudinal Velocity   {dot{x}}   [m/s]
%   LatVel     - (n,1 numeric) Lateral Velocity        {dot{y}}   [m/s]
%   YawVel     - (n,1 numeric) Yaw Velocity            {dot{psi}} [rad/s]
%
% Outputs:
%   LongAcc    - (n,1 numeric) Longitudinal Acceleration       {ddot{x}}  [m/s^2]
%   LatAcc     - (n,1 numeric) Lateral Acceleration            {ddot{y}}  [m/s^2]
%   YawAcc     - (n,1 numeric) Yaw Acceleration                {ddot{psi} [rad/s^2]
%   LongAccTot - (n,1 numeric) Total Longitudinal Acceleration {a_x}      [m/s^2]
%   LatAccTot  - (n,1 numeric) Total Lateral Acceleration      {a_y}      [m/s^2]
%
% Notes:
% check for correct yaw acc implementation
% Itterations need to be checked for rotational accelerations, like tire
% forces and yaw moments at each tire
% How do we solve for all suspension parameters, and how do they change
% over time
% Test Case fix
% Vertical Acc Parameters fix, understanding ride and implementing it
% IXX and IYY from CAD
% Array operations
%
% Author(s): 
% Tristan Pham       (atlpham@ucdavis.edu)        [Oct 2020 - ???     ]
% 
% Last Updated: 7-May-2022

%% Test Case
if nargin == 0
    TFx = zeros(1,4);
    TFy = [250, 250, 0, 0];
    TMz = zeros(1,4);
    
    AFx = -100;
    AFy = 0;
    AMz = 0;
    AFz = 0;
    AMy = 0;
    
    Wheelbase  = 1.575; 
    TrackWidth = 1.22;               %*ones(1,2); (FIXME)did a quick fix for array sizes 
    TrackWidthTest = 1.22*ones(1,2);
    Steer      = [18, 15, 1, -1];
    
    Mass         = 275;   
    YawInertia   = 130; 
    CoG          = [(0.47-0.5)*Wheelbase, 0, 0.25];
    PercentFront = 0.5;
    Sprung_COG_Height = 0;
    
    LongVel = 15;
    LatVel  = 0;
    YawVel  = 0.5;

    Front_View_Suspension_Arm = 0;   %calculation
    Side_View_Suspension_Arm = 0;
    Front_View_Jacking_Angle = 0;    
    Side_View_Jacking_Angle = 0;    
    
    Front_Roll_Stiffness = 0;
    Rear_Roll_Stiffness = 0;
    Roll_Dampening_Coeff_Front = 0;
    Roll_Dampening_Coeff_Rear = 0;
    Roll_Speed = 0;
    Roll = 0;

    Pitch_Stiffness = 0;
    Pitch_Dampening = 0;
    Pitch = 0;
    Pitch_Velocity = 0;

    Ride_Stiffness = 0;
    Ride = 0;
    Ride_Dampening = 0;
    Ride_Velocity = 0;

    Iyy = 0;
    Ixx = 0;

    z = 0;
    
    [LongAcc, LatAcc, YawAcc, LongAccTot, LatAccTot, VertAcc, RollAcc, PitchAcc] = ...
    ForceBasedRollCenter6DOFAccelerations( TFx, TFy, TMz, AFx, AFy, AMy, AMz, AFz, ...      
        Wheelbase, TrackWidth, TrackWidthTest, Steer, PercentFront, ...                      
        Front_View_Suspension_Arm, z, Side_View_Suspension_Arm, Front_View_Jacking_Angle, ...
        Side_View_Jacking_Angle, ...
        Front_Roll_Stiffness, Rear_Roll_Stiffness, Roll_Dampening_Coeff_Front, ...
        Roll_Dampening_Coeff_Rear, Roll_Speed, Roll, ...
        Pitch_Stiffness, Pitch_Dampening, Pitch, Pitch_Velocity, ...
        Ride_Stiffness, Ride, Ride_Dampening, Ride_Velocity,...
        Mass, YawInertia, CoG, Sprung_COG_Height, ...                                      
        LongVel, LatVel, YawVel, Ixx, Iyy)                    
    
    return;
end

%% Computations

%%% Tire Positions (n,4,3 numeric)
TirePos = cat( 3, Wheelbase/2 + [-1, -1, 1, 1].*CoG(:,1), ...
          [TrackWidthTest(:,1).*[1 -1]/2, TrackWidthTest(:,2).*[1 -1]/2], ...
          zeros( size(Steer) ) );

%%% Tire Loads (n,4,3 numeric)
TireLoad = cat( 3, TFx, TFy, zeros( size(Steer) ) );

%%% Tire Yaw Moment (n,1 numeric)
TireMoment = cross(TirePos, TireLoad, 3);
TMz = sum( TireMoment(:,:,3) ) + sum(TMz,2);

%%%Wheelbase Calculations
a = Wheelbase .* (1-PercentFront);
b = Wheelbase .* PercentFront;

%%%Chassis Accelerations

%%Yaw Acceleration
%Note: in overleaf there is the option of a or b

YawComputation1 = sum((TFx .* cosd(Steer) - TFy .* sind(Steer)) .* -TrackWidth ./ 2 ...
    + (TFx .* sind(Steer) + TFy .* cosd(Steer)) .* (a) + TMz);

YawComputation2 = sum((TFx .* cosd(Steer) - TFy .* sind(Steer)) .* TrackWidth ./ 2 ...
    + (TFx .* sind(Steer) + TFy .* cosd(Steer)) .* (a) + TMz);

YawAcc = ((YawComputation1 + YawComputation2) - AFy .* (Wheelbase ./ 2 - a) - AMz) ./ YawInertia;

%%Roll Acceleration 
% What to put for z
RollAcc = (sum((TFx .* sind(Steer) + TFy .* cosd(Steer)) .* Front_View_Suspension_Arm...
    - (TFx .* cosd(Steer) - TFy .* sind(Steer)) .* tand(Side_View_Jacking_Angle) .* TrackWidth ./ 2)...
    - AFy .* (Sprung_COG_Height + z) - AMz - (Front_Roll_Stiffness + Rear_Roll_Stiffness) .* Roll...
    - (Roll_Dampening_Coeff_Front + Roll_Dampening_Coeff_Rear) .* Roll_Speed) ./ Ixx;

%%Pitch Acceleration
%Note* in overleaf there is the option of a or b
PitchAcc = (sum(-(TFx .* cosd(Steer) - TFy .* sind(Steer)) .* Side_View_Suspension_Arm...
    + (TFx .* sind(Steer) + TFy .* cosd(Steer)) .* tand(Front_View_Jacking_Angle).* (a) )...
    + AFx .* (Sprung_COG_Height + z) - AFz .* (a - Wheelbase ./ 2) - AMy ...
    - Pitch_Stiffness .* Pitch - Pitch_Dampening .* Pitch_Velocity) ./ Iyy;


%%Longitudinal Acceleration
LongAcc = ((sum( TFx.*cosd(Steer) - TFy.*sind(Steer), 2 ) - AFx) ./ Mass) + LatVel.*YawVel;

%%Lateral Acceleration
LatAcc  = ((sum( TFy.*cosd(Steer) + TFx.*sind(Steer), 2 ) - AFy) ./ Mass) - LongVel.*YawVel;

%%Vertical Acceleration
VertAcc = (sum(Ride_Stiffness .* Ride + Ride_Dampening .* Ride_Velocity + (TFx .* cosd(Steer) - TFy .* sind(Steer)) .* tand(Side_View_Jacking_Angle)...
    + (TFy .* cosd(Steer) + TFx .* sind(Steer)) .* tan(Front_View_Jacking_Angle)) - AFz) ./ Mass;

LongAccTot = LongAcc - LatVel .*YawVel;
LatAccTot  = LatAcc  + LongVel.*YawVel;
